simulink model "HEV_Simu_V1_1_RT"  (R2018a)
settings: Solver=ode23s  StartTime=0.0  StopTime=660  FixedStep=0.001  EnableMultiTasking=on
PreLoadFcn:
  | HevSimuVccWs_V1_PreLoad
StartFcn:
  | tic
StopFcn:
  | toc
  | disp(['実時間の' num2str(max(tout)/toc) '倍速'])
model workspace (MAT data in the model file):
  Var = 0
undefined symbols (not defined in the file or in its folder): canChannel
libraries: canmsglib x55, canlib x35, simulink x2, sldrtlib x1
(part 3 of 4)

== system HEV_Simu_V1_1_RT/Controller/CtrlStrct_VNT_Level_2/VNT_Level_2_CAN/Motor_Ctrl/MotorCtrl_PwtrCAN Tx ==
  note: Function of CAN transmit
      | ・conversion fromCAN application signal to signal of CAN message
  note: Motor Control
  note: CAN transmit
  IMotorCtrl_PwtrCAN_Tx_Apli : Inport
  Bus Creator1 : BusCreator  Inputs=1
  Bus Selector1 : BusSelector  OutputSignals=MtrCtrl_Motor_regen_torque_available,MtrCtrl_Motor_torque_actual,MtrCtrl_Motor_torque_available
  MotorCtrl_PwtrCAN Pack : canmsglib/CAN Pack  CANdbFile=HEV_CANDB.dbc  MsgList=MotorCtrl_PwtrCAN_Tx  MsgName=MotorCtrl_PwtrCAN_Tx  MsgIDType=Extended (29-bit identifier)  MsgIdentifier=218058883  MsgLength=8  SignalInfo=MtrCtrl_Motor_regen_torque_avail$32$16$1$1$1$0$1.000000e-02$0$-300$300$#MtrCtrl_Motor_torque_actual$0$16$1$1$1$0$1.000000e-02$0$-300$300$#MtrCtrl_Motor_torque_available$16$16$1$1$1$0$1.000000e-02$0$-300$300$#  NSignals=3  StartBits=str2num('[int32(32);int32(0);int32(16)]')  SignalSizes=str2num('[int32(16);int32(16);int32(16)]')  ByteOrders=str2num('[int32(1);int32(1);int32(1)]')  DataTypes=str2num('[int32(1);int32(1);int32(1)]')  MultiplexTypes=str2num('[int32(1);int32(1);int32(1)]')  MultiplexValues=str2num('[double(0);double(0);double(0)]')  Factors=str2num('[double(1.000000e-02);double(1.000000e-02);double(1.000000e-02)]')  Offsets=str2num('[double(0);double(0);double(0)]')  Minimums=str2num('[double(-300);double(-300);double(-300)]')  Maximums=str2num('[double(300);double(300);double(300)]')  Remote=off  ApplyMinMax=off  BusOutput=off
      settings: AttributesFormatString=<CANdbFile = %<CANdbFile>>  SourceProductName=Simulink Real-Time  SourceProductBaseCode=XP  DataFormat=CANdb specified signals
  MotorCtrl_PwtrCAN Transmit : canlib/CAN Transmit  BlockHandle=19377.0016  DeviceMenu=Vector CANcaseXL 1 (Channel 1)  Device=Vector CANcaseXL 1 (Channel 1)  ObjConstructor=canChannel('Vector','CANcaseXL 1',1)  EnablePeriodicTransmit=on  MessagePeriod=0.01
      settings: AttributesFormatString=<MessagePeriod = %<MessagePeriod>>  SourceProductName=Vehicle Network Toolbox  SourceProductBaseCode=VN
  MotorCtrl_PwtrCAN_Tx_0CFF5083 : Outport
  wires:
  Bus Selector1/2 -> MotorCtrl_PwtrCAN Pack/2  "<MtrCtrl_Motor_torque_actual>"
  Bus Creator1/1 -> MotorCtrl_PwtrCAN Transmit/1, MotorCtrl_PwtrCAN_Tx_0CFF5083/1  "MotorCtrl_PwtrCAN_Tx"
  Bus Selector1/3 -> MotorCtrl_PwtrCAN Pack/3  "<MtrCtrl_Motor_torque_available>"
  MotorCtrl_PwtrCAN Pack/1 -> Bus Creator1/1  "MotorCtrl_PwtrCAN_Tx_0CFF5083"
  IMotorCtrl_PwtrCAN_Tx_Apli/1 -> Bus Selector1/1
  Bus Selector1/1 -> MotorCtrl_PwtrCAN Pack/1  "<MtrCtrl_Motor_regen_torque_available>"

== system HEV_Simu_V1_1_RT/Controller/CtrlStrct_VNT_Level_2/VNT_Level_2_CAN/Motor_Ctrl/MotorCtrl_PwtrCAN_Rx ==
  note: Function of CAN receive
      | ・CAN message selection
      | ・conversion from CAN signal to CAN application signal with bus object
  note: Motor Control
  note: CAN receive
  PwtrCAN : Inport
  Bus Creator7 : BusCreator  Inputs=3
  Bus Selector3 : BusSelector  OutputSignals=HEV_Ctrl_PwtrCAN_Tx_0CFF2082
  Bus Selector4 : BusSelector  OutputSignals=EngineCtrl_PwtrCAN_Tx_0CFF3000
  Bus Selector5 : BusSelector  OutputSignals=TransmCtrl_PwtrCAN_Tx_0CFF4003
  MotorCtrl_PwtrCAN Receive : canlib/CAN Receive  BlockHandle=19439.0016  DeviceMenu=Vector CANcaseXL 1 (Channel 2)  Device=Vector CANcaseXL 1 (Channel 2)  ObjConstructor=canChannel('Vector','CANcaseXL 1',2)  EnableStandardIDsFilter=off  StandardIDs=0  EnableExtendedIDsFilter=off  ExtendedIDs=0  SampleTime=0.01  MsgsPerTimestep=all  StdIDsCombo=Allow all  ExtIDsCombo=Allow all  InternalFilterUpdateStatus=on  BusOutput=off
      settings: AttributesFormatString=<SampleTime = %<SampleTime>>  SourceProductName=Vehicle Network Toolbox  SourceProductBaseCode=VN
  MotorCtrl_PwtrCAN_Receive_10ms : Subsystem
  Rate Transition1 : RateTransition  Deterministic=off
      settings: AttributesFormatString=<Deterministic=%<Deterministic>>
  Terminator : Terminator
  Terminator1 : Terminator
  Terminator2 : Terminator
  MotorCtrl_PwtrCAN_Rx : Outport
  wires:
  PwtrCAN/1 -> Bus Selector4/1, Bus Selector3/1, Bus Selector5/1
  Bus Creator7/1 -> Rate Transition1/1
  Rate Transition1/1 -> MotorCtrl_PwtrCAN_Rx/1  "MotorCtrl_PwtrCAN_Rx"
  Bus Selector5/1 -> Terminator/1  "<TransmCtrl_PwtrCAN_Tx_0CFF4003>"
  Bus Selector3/1 -> Terminator1/1  "<HEV_Ctrl_PwtrCAN_Tx_0CFF2082>"
  Bus Selector4/1 -> Terminator2/1  "<EngineCtrl_PwtrCAN_Tx_0CFF3000>"
  MotorCtrl_PwtrCAN_Receive_10ms/1(TmCtrl_Clutch_position) -> Bus Creator7/1
  MotorCtrl_PwtrCAN_Receive_10ms/2(HEVCtrl_Motor_torque_request) -> Bus Creator7/2
  MotorCtrl_PwtrCAN_Receive_10ms/3(EngCtrl_Engine_speed) -> Bus Creator7/3
  MotorCtrl_PwtrCAN Receive/2 -> MotorCtrl_PwtrCAN_Receive_10ms/1(PwtrCAN_Msg)
  MotorCtrl_PwtrCAN Receive/1 -> MotorCtrl_PwtrCAN_Receive_10ms/Trigger

== system HEV_Simu_V1_1_RT/Controller/CtrlStrct_VNT_Level_2/VNT_Level_2_CAN/NAVI/NAVI_CAN_Rx ==
  note: CAN receive
  note: Navigation
  InfoCAN : Inport
  Bus Creator : BusCreator  Inputs=1  OutDataTypeStr=Bus: NAVI_InfoCAN_Rx_Bus
      settings: AttributesFormatString=<%<OutDataTypeStr>>
  Bus Selector1 : BusSelector  OutputSignals=Gateway_InfoCAN_Tx_0CFFC485
  NAVI_InfoCAN Receive : canlib/CAN Receive  BlockHandle=19512.0016  DeviceMenu=Vector CANcaseXL 1 (Channel 2)  Device=Vector CANcaseXL 1 (Channel 2)  ObjConstructor=canChannel('Vector','CANcaseXL 1',2)  EnableStandardIDsFilter=off  StandardIDs=0  EnableExtendedIDsFilter=off  ExtendedIDs=0  SampleTime=0.1  MsgsPerTimestep=all  StdIDsCombo=Allow all  ExtIDsCombo=Allow all  InternalFilterUpdateStatus=on  BusOutput=off
      settings: AttributesFormatString=<SampleTime = %<SampleTime>>  SourceProductName=Vehicle Network Toolbox  SourceProductBaseCode=VN
  NAVI_InfoCAN_Receive_100ms : Subsystem
  Rate Transition1 : RateTransition  Deterministic=off
      settings: AttributesFormatString=<Deterministic=%<Deterministic>>
  Terminator : Terminator
  NAVI_InfoCAN_Rx : Outport
  wires:
  Rate Transition1/1 -> NAVI_InfoCAN_Rx/1  "NAVI_InfoCAN_Rx"
  InfoCAN/1 -> Bus Selector1/1
  Bus Selector1/1 -> Terminator/1  "<Gateway_InfoCAN_Tx_0CFFC485>"
  NAVI_InfoCAN Receive/2 -> NAVI_InfoCAN_Receive_100ms/1(InfoCAN_Msg)
  NAVI_InfoCAN Receive/1 -> NAVI_InfoCAN_Receive_100ms/Trigger
  Bus Creator/1 -> Rate Transition1/1
  NAVI_InfoCAN_Receive_100ms/1(BrkCtrl_Vehicle_speed) -> Bus Creator/1

== system HEV_Simu_V1_1_RT/Controller/CtrlStrct_VNT_Level_2/VNT_Level_2_CAN/NAVI/NAVI_CAN_Tx ==
  note: CAN transmit
  note: Navigation
  NAVI_InfoCAN_Tx_Apli : Inport
  Bus Creator1 : BusCreator  Inputs=1
  Bus Selector3 : BusSelector  OutputSignals=NAVI_Home_around_status,NAVI_Road_information
  NAVI_InfoCAN Pack : canmsglib/CAN Pack  CANdbFile=HEV_CANDB.dbc  MsgList=NAVI_InfoCAN_Tx  MsgName=NAVI_InfoCAN_Tx  MsgIDType=Extended (29-bit identifier)  MsgIdentifier=218083356  MsgLength=8  SignalInfo=NAVI_Home_around_status$16$16$1$2$1$0$1$0$0$65535$#NAVI_Road_information$0$16$1$2$1$0$1$0$0$65535$#  NSignals=2  StartBits=str2num('[int32(16);int32(0)]')  SignalSizes=str2num('[int32(16);int32(16)]')  ByteOrders=str2num('[int32(1);int32(1)]')  DataTypes=str2num('[int32(2);int32(2)]')  MultiplexTypes=str2num('[int32(1);int32(1)]')  MultiplexValues=str2num('[double(0);double(0)]')  Factors=str2num('[double(1);double(1)]')  Offsets=str2num('[double(0);double(0)]')  Minimums=str2num('[double(0);double(0)]')  Maximums=str2num('[double(65535);double(65535)]')  Remote=off  ApplyMinMax=off  BusOutput=off
      settings: AttributesFormatString=<CANdbFile = %<CANdbFile>>  SourceProductName=Simulink Real-Time  SourceProductBaseCode=XP  DataFormat=CANdb specified signals
  NAVI_InfoCAN Transmit : canlib/CAN Transmit  BlockHandle=20931.0017  DeviceMenu=Vector CANcaseXL 1 (Channel 1)  Device=Vector CANcaseXL 1 (Channel 1)  ObjConstructor=canChannel('Vector','CANcaseXL 1',1)  EnablePeriodicTransmit=on  MessagePeriod=0.1
      settings: AttributesFormatString=<MessagePeriod = %<MessagePeriod>>  SourceProductName=Vehicle Network Toolbox  SourceProductBaseCode=VN
  NAVI_InfoCAN_Tx : Outport
  wires:
  Bus Creator1/1 -> NAVI_InfoCAN_Tx/1  "NAVI_InfoCAN_Tx"
  Bus Selector3/1 -> NAVI_InfoCAN Pack/1  "<NAVI_Home_around_status>"
  NAVI_InfoCAN Pack/1 -> NAVI_InfoCAN Transmit/1, Bus Creator1/1  "NAVI_InfoCAN_Tx_0CFFB01C"
  Bus Selector3/2 -> NAVI_InfoCAN Pack/2  "<NAVI_Road_information>"
  NAVI_InfoCAN_Tx_Apli/1 -> Bus Selector3/1

== system HEV_Simu_V1_1_RT/Controller/CtrlStrct_VNT_Level_2/VNT_Level_2_CAN/Radar/Radar_CAN_Rx ==
  note: Function of CAN receive
      | ・CAN message selection
      | ・conversion from CAN signal to CAN application signal with bus object
  note: Radar Detection
  note: CAN receive
  InfoCAN : Inport
  Bus Creator : BusCreator  Inputs=1
  Bus Selector1 : BusSelector  OutputSignals=Gateway_InfoCAN_Tx_0CFFC485
  Radar_InfoCAN Receive : canlib/CAN Receive  BlockHandle=20997.0016  DeviceMenu=Vector CANcaseXL 1 (Channel 2)  Device=Vector CANcaseXL 1 (Channel 2)  ObjConstructor=canChannel('Vector','CANcaseXL 1',2)  EnableStandardIDsFilter=off  StandardIDs=0  EnableExtendedIDsFilter=off  ExtendedIDs=0  SampleTime=0.1  MsgsPerTimestep=all  StdIDsCombo=Allow all  ExtIDsCombo=Allow all  InternalFilterUpdateStatus=on  BusOutput=off
      settings: AttributesFormatString=<SampleTime = %<SampleTime>>  SourceProductName=Vehicle Network Toolbox  SourceProductBaseCode=VN
  Radar_InfoCAN_Receive_100ms : Subsystem
  Rate Transition1 : RateTransition  Deterministic=off
      settings: AttributesFormatString=<Deterministic=%<Deterministic>>
  Terminator : Terminator
  Radar_InfoCAN_Rx : Outport
  wires:
  Rate Transition1/1 -> Radar_InfoCAN_Rx/1  "Radar_InfoCAN_Rx"
  Bus Creator/1 -> Rate Transition1/1
  InfoCAN/1 -> Bus Selector1/1
  Bus Selector1/1 -> Terminator/1  "<Gateway_InfoCAN_Tx_0CFFC485>"
  Radar_InfoCAN_Receive_100ms/1(BrkCtrl_Vehicle_speed) -> Bus Creator/1
  Radar_InfoCAN Receive/2 -> Radar_InfoCAN_Receive_100ms/1(InfoCAN_Msg)
  Radar_InfoCAN Receive/1 -> Radar_InfoCAN_Receive_100ms/Trigger

== system HEV_Simu_V1_1_RT/Controller/CtrlStrct_VNT_Level_2/VNT_Level_2_CAN/Radar/Radar_CAN_Tx ==
  note: Radar Detection
  note: CAN transmit
  note: Function of CAN transmit
      | ・conversion fromCAN application signal to signal of CAN message
  Radar_InfoCAN_Tx_Apli : Inport
  Bus Creator1 : BusCreator  Inputs=1
  Bus Selector3 : BusSelector  OutputSignals=Radar_Relative_distance,Radar_Relative_velocity
  Radar_InfoCAN Pack : canmsglib/CAN Pack  CANdbFile=HEV_CANDB.dbc  MsgList=Radar_InfoCAN_Tx  MsgName=Radar_InfoCAN_Tx  MsgIDType=Extended (29-bit identifier)  MsgIdentifier=218038400  MsgLength=8  SignalInfo=Radar_Relative_distance$0$16$1$2$1$0$1.000000e-02$0$0$500$#Radar_Relative_velocity$16$16$1$1$1$0$1.000000e-02$0$-50$50$#  NSignals=2  StartBits=str2num('[int32(0);int32(16)]')  SignalSizes=str2num('[int32(16);int32(16)]')  ByteOrders=str2num('[int32(1);int32(1)]')  DataTypes=str2num('[int32(2);int32(1)]')  MultiplexTypes=str2num('[int32(1);int32(1)]')  MultiplexValues=str2num('[double(0);double(0)]')  Factors=str2num('[double(1.000000e-02);double(1.000000e-02)]')  Offsets=str2num('[double(0);double(0)]')  Minimums=str2num('[double(0);double(-50)]')  Maximums=str2num('[double(500);double(50)]')  Remote=off  ApplyMinMax=off  BusOutput=off
      settings: AttributesFormatString=<CANdbFile = %<CANdbFile>>  SourceProductName=Simulink Real-Time  SourceProductBaseCode=XP  DataFormat=CANdb specified signals
  Radar_InfoCAN Transmit : canlib/CAN Transmit  BlockHandle=21025.0016  DeviceMenu=Vector CANcaseXL 1 (Channel 1)  Device=Vector CANcaseXL 1 (Channel 1)  ObjConstructor=canChannel('Vector','CANcaseXL 1',1)  EnablePeriodicTransmit=on  MessagePeriod=0.1
      settings: AttributesFormatString=<MessagePeriod = %<MessagePeriod>>  SourceProductName=Vehicle Network Toolbox  SourceProductBaseCode=VN
  Radar_InfoCAN_Tx : Outport
  wires:
  Bus Creator1/1 -> Radar_InfoCAN_Tx/1  "Radar_InfoCAN_Tx"
  Radar_InfoCAN_Tx_Apli/1 -> Bus Selector3/1
  Radar_InfoCAN Pack/1 -> Bus Creator1/1, Radar_InfoCAN Transmit/1  "Radar_InfoCAN_Tx_0CFF0080"
  Bus Selector3/2 -> Radar_InfoCAN Pack/2  "<Radar_Relative_velocity>"
  Bus Selector3/1 -> Radar_InfoCAN Pack/1  "<Radar_Relative_distance>"

== system HEV_Simu_V1_1_RT/Controller/CtrlStrct_VNT_Level_2/VNT_Level_2_CAN/Steer_Ctrl/SteerCtrl_VehCAN Tx ==
  note: Steering Control
  note: Function of CAN transmit
      | ・conversion fromCAN application signal to signal of CAN message
  note: CAN transmit
  SteerCtrl_VehCAN_Tx_Apli : Inport
  Bus Creator1 : BusCreator  Inputs=1
  Bus Selector1 : BusSelector  OutputSignals=StrgCtrl_Steer_angle
  SteerCtrl_VehCAN Pack : canmsglib/CAN Pack  CANdbFile=HEV_CANDB.dbc  MsgList=SteerCtrl_VehCAN_Tx  MsgName=SteerCtrl_VehCAN_Tx  MsgIDType=Extended (29-bit identifier)  MsgIdentifier=218066963  MsgLength=8  SignalInfo=StrgCtrl_Steer_angle$0$16$1$1$1$0$3.125000e-02$0$-720$720$#  NSignals=1  StartBits=str2num('[int32(0)]')  SignalSizes=str2num('[int32(16)]')  ByteOrders=str2num('[int32(1)]')  DataTypes=str2num('[int32(1)]')  MultiplexTypes=str2num('[int32(1)]')  MultiplexValues=str2num('[double(0)]')  Factors=str2num('[double(3.125000e-02)]')  Offsets=str2num('[double(0)]')  Minimums=str2num('[double(-720)]')  Maximums=str2num('[double(720)]')  Remote=off  ApplyMinMax=off  BusOutput=off
      settings: AttributesFormatString=<CANdbFile = %<CANdbFile>>  SourceProductName=Simulink Real-Time  SourceProductBaseCode=XP  DataFormat=CANdb specified signals
  SteerCtrl_VehCAN Transmit : canlib/CAN Transmit  BlockHandle=21054.0016  DeviceMenu=Vector CANcaseXL 1 (Channel 1)  Device=Vector CANcaseXL 1 (Channel 1)  ObjConstructor=canChannel('Vector','CANcaseXL 1',1)  EnablePeriodicTransmit=on  MessagePeriod=0.05
      settings: AttributesFormatString=<MessagePeriod = %<MessagePeriod>>  SourceProductName=Vehicle Network Toolbox  SourceProductBaseCode=VN
  SteerCtrl_VehCAN_Tx : Outport
  wires:
  SteerCtrl_VehCAN Pack/1 -> SteerCtrl_VehCAN Transmit/1, Bus Creator1/1  "SteerCtrl_VehCAN_Tx_0CFF7013"
  Bus Selector1/1 -> SteerCtrl_VehCAN Pack/1  "<StrgCtrl_Steer_angle>"
  SteerCtrl_VehCAN_Tx_Apli/1 -> Bus Selector1/1
  Bus Creator1/1 -> SteerCtrl_VehCAN_Tx/1  "SteerCtrl_VehCAN_Tx"

== system HEV_Simu_V1_1_RT/Controller/CtrlStrct_VNT_Level_2/VNT_Level_2_CAN/Steer_Ctrl/SteerCtrl_VehCAN_Rx ==
  note: Steering Control
  note: Function of CAN receive
      | ・CAN message selection
      | ・conversion from CAN signal to CAN application signal with bus object
  note: CAN receive
  In1 : Inport
  Bus Creator : BusCreator  Inputs=1
  Bus Selector7 : BusSelector  OutputSignals=BrakeCtrl_VehCAN_Tx_0CFF600B
  Rate Transition1 : RateTransition  Deterministic=off
      settings: AttributesFormatString=<Deterministic=%<Deterministic>>
  SteerCtrl_VehCAN Receive : canlib/CAN Receive  BlockHandle=21070.0016  DeviceMenu=Vector CANcaseXL 1 (Channel 2)  Device=Vector CANcaseXL 1 (Channel 2)  ObjConstructor=canChannel('Vector','CANcaseXL 1',2)  EnableStandardIDsFilter=off  StandardIDs=0  EnableExtendedIDsFilter=off  ExtendedIDs=0  SampleTime=0.05  MsgsPerTimestep=all  StdIDsCombo=Allow all  ExtIDsCombo=Allow all  InternalFilterUpdateStatus=on  BusOutput=off
      settings: AttributesFormatString=<SampleTime = %<SampleTime>>  SourceProductName=Vehicle Network Toolbox  SourceProductBaseCode=VN
  SteerCtrl_VehCAN_Receive50ms : Subsystem
  Terminator : Terminator
  SteerCtrl_VehCAN_Rx : Outport
  wires:
  In1/1 -> Bus Selector7/1
  Bus Creator/1 -> Rate Transition1/1
  Rate Transition1/1 -> SteerCtrl_VehCAN_Rx/1  "SteerCtrl_VehCAN_Rx"
  Bus Selector7/1 -> Terminator/1  "<BrakeCtrl_VehCAN_Tx_0CFF600B>"
  SteerCtrl_VehCAN_Receive50ms/1(BrkCtrl_Vehicle_speed) -> Bus Creator/1
  SteerCtrl_VehCAN Receive/1 -> SteerCtrl_VehCAN_Receive50ms/Trigger
  SteerCtrl_VehCAN Receive/2 -> SteerCtrl_VehCAN_Receive50ms/1(VehCAN_Msg)

== system HEV_Simu_V1_1_RT/Controller/CtrlStrct_VNT_Level_2/VNT_Level_2_CAN/Transms_Ctrl/TransmCtrl_PwtrCAN Tx ==
  note: Function of CAN transmit
      | ・conversion fromCAN application signal to signal of CAN message
  note: Transmission Control
  note: CAN transmit
  TransmCtrl_PwtrCAN_Tx_Apli : Inport
  Bus Creator1 : BusCreator  Inputs=1
  Bus Selector2 : BusSelector  OutputSignals=TmCtrl_Clutch_position,TmCtrl_Gear_position
  TransmCtrl_PwtrCAN Pack : canmsglib/CAN Pack  CANdbFile=HEV_CANDB.dbc  MsgList=TransmCtrl_PwtrCAN_Tx  MsgName=TransmCtrl_PwtrCAN_Tx  MsgIDType=Extended (29-bit identifier)  MsgIdentifier=218054659  MsgLength=8  SignalInfo=TmCtrl_Clutch_position$0$8$1$2$1$0$1.000000e-02$0$0$1$#TmCtrl_Gear_position$8$8$1$2$1$0$1$0$0$5$#  NSignals=2  StartBits=str2num('[int32(0);int32(8)]')  SignalSizes=str2num('[int32(8);int32(8)]')  ByteOrders=str2num('[int32(1);int32(1)]')  DataTypes=str2num('[int32(2);int32(2)]')  MultiplexTypes=str2num('[int32(1);int32(1)]')  MultiplexValues=str2num('[double(0);double(0)]')  Factors=str2num('[double(1.000000e-02);double(1)]')  Offsets=str2num('[double(0);double(0)]')  Minimums=str2num('[double(0);double(0)]')  Maximums=str2num('[double(1);double(5)]')  Remote=off  ApplyMinMax=off  BusOutput=off
      settings: AttributesFormatString=<CANdbFile = %<CANdbFile>>  SourceProductName=Simulink Real-Time  SourceProductBaseCode=XP  DataFormat=CANdb specified signals
  TransmCtrl_PwtrCAN Transmit : canlib/CAN Transmit  BlockHandle=21269.0016  DeviceMenu=Vector CANcaseXL 1 (Channel 1)  Device=Vector CANcaseXL 1 (Channel 1)  ObjConstructor=canChannel('Vector','CANcaseXL 1',1)  EnablePeriodicTransmit=on  MessagePeriod=0.01
      settings: AttributesFormatString=<MessagePeriod = %<MessagePeriod>>  SourceProductName=Vehicle Network Toolbox  SourceProductBaseCode=VN
  TransmCtrl_PwtrCAN_Tx : Outport
  wires:
  TransmCtrl_PwtrCAN_Tx_Apli/1 -> Bus Selector2/1
  TransmCtrl_PwtrCAN Pack/1 -> Bus Creator1/1  "TransmCtrl_PwtrCAN_Tx_0CFF4003"
  Bus Creator1/1 -> TransmCtrl_PwtrCAN Transmit/1, TransmCtrl_PwtrCAN_Tx/1  "TransmCtrl_PwtrCAN_Tx"
  Bus Selector2/2 -> TransmCtrl_PwtrCAN Pack/2  "<TmCtrl_Gear_position>"
  Bus Selector2/1 -> TransmCtrl_PwtrCAN Pack/1  "<TmCtrl_Clutch_position>"

== system HEV_Simu_V1_1_RT/Controller/CtrlStrct_VNT_Level_2/VNT_Level_2_CAN/Transms_Ctrl/TransmCtrl_PwtrCAN_Rx ==
  note: Transmission Control
  note: Function of CAN receive
      | ・CAN message selection
      | ・conversion from CAN signal to CAN application signal with bus object
  note: CAN receive
  PwtrCAN : Inport
  Bus Creator6 : BusCreator  Inputs=2
  Bus Selector3 : BusSelector  OutputSignals=EngineCtrl_PwtrCAN_Tx_0CFF3000
  Bus Selector7 : BusSelector  OutputSignals=Gateway_PwtrCAN_Tx_0CFFC385
  Rate Transition1 : RateTransition  Deterministic=off
      settings: AttributesFormatString=<Deterministic=%<Deterministic>>
  Terminator : Terminator
  Terminator1 : Terminator
  TransmCtrl_PwtrCAN Receive : canlib/CAN Receive  BlockHandle=23424.0016  DeviceMenu=Vector CANcaseXL 1 (Channel 2)  Device=Vector CANcaseXL 1 (Channel 2)  ObjConstructor=canChannel('Vector','CANcaseXL 1',2)  EnableStandardIDsFilter=off  StandardIDs=0  EnableExtendedIDsFilter=off  ExtendedIDs=0  SampleTime=0.01  MsgsPerTimestep=all  StdIDsCombo=Allow all  ExtIDsCombo=Allow all  InternalFilterUpdateStatus=on  BusOutput=off
      settings: AttributesFormatString=<SampleTime = %<SampleTime>>  SourceProductName=Vehicle Network Toolbox  SourceProductBaseCode=VN
  TransmCtrl_PwtrCAN_Receive_10ms : Subsystem
  TransmCtrl_PwtrCAN_Rx : Outport
  wires:
  PwtrCAN/1 -> Bus Selector3/1, Bus Selector7/1
  Rate Transition1/1 -> TransmCtrl_PwtrCAN_Rx/1  "TransmCtrl_PwtrCAN_Rx"
  Bus Creator6/1 -> Rate Transition1/1
  Bus Selector7/1 -> Terminator/1  "<Gateway_PwtrCAN_Tx_0CFFC385>"
  Bus Selector3/1 -> Terminator1/1  "<EngineCtrl_PwtrCAN_Tx_0CFF3000>"
  TransmCtrl_PwtrCAN_Receive_10ms/1(BrkCtrl_Vehicle_speed) -> Bus Creator6/1
  TransmCtrl_PwtrCAN_Receive_10ms/2(EngCtrl_Engine_speed) -> Bus Creator6/2
  TransmCtrl_PwtrCAN Receive/1 -> TransmCtrl_PwtrCAN_Receive_10ms/Trigger
  TransmCtrl_PwtrCAN Receive/2 -> TransmCtrl_PwtrCAN_Receive_10ms/1(PwtrCAN_Msg)

== system HEV_Simu_V1_1_RT/Controller/CtrlStrct_VNT_Level_2/VNT_Level_2_CAN/VM_Ctrl/VM_Ctrl_VehCAN Tx ==
  note: Vehicle Motion Control
  note: Function of CAN transmit
      | ・conversion fromCAN application signal to signal of CAN message
  note: CAN transmit
  VM_Ctrl_VehCAN_Tx_Apli : Inport
  Bus Creator1 : BusCreator  Inputs=1
  Bus Selector3 : BusSelector  OutputSignals=VMCtrl_BrakeForceCmnd,VMCtrl_BrakeForceStatus,VMCtrl_PropTorqCmnd,VMCtrl_PropTorqStatus
  VM_Ctrl_VehCAN Pack : canmsglib/CAN Pack  CANdbFile=HEV_CANDB.dbc  MsgList=VM_Ctrl_VehCAN_Tx  MsgName=VM_Ctrl_VehCAN_Tx  MsgIDType=Extended (29-bit identifier)  MsgIdentifier=218091654  MsgLength=8  SignalInfo=VMCtrl_BrakeTorqCmnd$32$16$1$1$1$0$1.000000e-02$0$-300$300$#VMCtrl_BrakeTorqStatus$24$8$1$2$1$0$1$0$0$7$#VMCtrl_PropTorqCmnd$8$16$1$1$1$0$1.000000e-02$0$-300$300$#VMCtrl_PropTorqStatus$0$8$1$2$1$0$1$0$-Inf$Inf$#  NSignals=4  StartBits=str2num('[int32(32);int32(24);int32(8);int32(0)]')  SignalSizes=str2num('[int32(16);int32(8);int32(16);int32(8)]')  ByteOrders=str2num('[int32(1);int32(1);int32(1);int32(1)]')  DataTypes=str2num('[int32(1);int32(2);int32(1);int32(2)]')  MultiplexTypes=str2num('[int32(1);int32(1);int32(1);int32(1)]')  MultiplexValues=str2num('[double(0);double(0);double(0);double(0)]')  Factors=str2num('[double(1.000000e-02);double(1);double(1.000000e-02);double(1)]')  Offsets=str2num('[double(0);double(0);double(0);double(0)]')  Minimums=str2num('[double(-300);double(0);double(-300);double(-Inf)]')  Maximums=str2num('[double(300);double(7);double(300);double(Inf)]')  Remote=off  ApplyMinMax=off  BusOutput=off
      settings: AttributesFormatString=<CANdbFile = %<CANdbFile>>  SourceProductName=Simulink Real-Time  SourceProductBaseCode=XP  DataFormat=CANdb specified signals
  VM_Ctrl_VehCAN Transmit : canlib/CAN Transmit  BlockHandle=26337.0018  DeviceMenu=Vector CANcaseXL 1 (Channel 1)  Device=Vector CANcaseXL 1 (Channel 1)  ObjConstructor=canChannel('Vector','CANcaseXL 1',1)  EnablePeriodicTransmit=on  MessagePeriod=0.05
      settings: AttributesFormatString=<MessagePeriod = %<MessagePeriod>>  SourceProductName=Vehicle Network Toolbox  SourceProductBaseCode=VN
  VM_Ctrl_VehCAN_Tx : Outport
  wires:
  Bus Selector3/1 -> VM_Ctrl_VehCAN Pack/1  "<VMCtrl_BrakeForceCmnd>"
  Bus Selector3/2 -> VM_Ctrl_VehCAN Pack/2  "<VMCtrl_BrakeForceStatus>"
  Bus Selector3/3 -> VM_Ctrl_VehCAN Pack/3  "<VMCtrl_PropTorqCmnd>"
  VM_Ctrl_VehCAN Pack/1 -> VM_Ctrl_VehCAN Transmit/1, Bus Creator1/1  "VM_Ctrl_VehCAN_Tx_0CFFD086"
  VM_Ctrl_VehCAN_Tx_Apli/1 -> Bus Selector3/1
  Bus Creator1/1 -> VM_Ctrl_VehCAN_Tx/1  "VM_Ctrl_VehCAN_Tx"
  Bus Selector3/4 -> VM_Ctrl_VehCAN Pack/4  "<VMCtrl_PropTorqStatus>"

== system HEV_Simu_V1_1_RT/Controller/CtrlStrct_VNT_Level_2/VNT_Level_2_CAN/VM_Ctrl/VM_Ctrl_VehCAN_Rx ==
  note: Vehicle Motion Control
  note: Function of CAN receive
      | ・CAN message selection
      | ・conversion from CAN signal to CAN application signal with bus object
  note: CAN receive
  In1 : Inport
  Bus Creator : BusCreator  Inputs=1
  Bus Selector7 : BusSelector  OutputSignals=BrakeCtrl_VehCAN_Tx_0CFF600B
  Rate Transition1 : RateTransition  Deterministic=off
      settings: AttributesFormatString=<Deterministic=%<Deterministic>>
  Terminator : Terminator
  VM_Ctrl_VehCAN Receive : canlib/CAN Receive  BlockHandle=26357.0018  DeviceMenu=Vector CANcaseXL 1 (Channel 2)  Device=Vector CANcaseXL 1 (Channel 2)  ObjConstructor=canChannel('Vector','CANcaseXL 1',2)  EnableStandardIDsFilter=off  StandardIDs=0  EnableExtendedIDsFilter=off  ExtendedIDs=0  SampleTime=0.05  MsgsPerTimestep=all  StdIDsCombo=Allow all  ExtIDsCombo=Allow all  InternalFilterUpdateStatus=on  BusOutput=off
      settings: AttributesFormatString=<SampleTime = %<SampleTime>>  SourceProductName=Vehicle Network Toolbox  SourceProductBaseCode=VN
  VM_Ctrl_VehCAN_Receive_50ms : Subsystem
  VM_Ctrl_VehCAN_Rx : Outport
  wires:
  Bus Creator/1 -> Rate Transition1/1
  Rate Transition1/1 -> VM_Ctrl_VehCAN_Rx/1  "VM_Ctrl_VehCAN_Rx"
  In1/1 -> Bus Selector7/1
  Bus Selector7/1 -> Terminator/1  "<BrakeCtrl_VehCAN_Tx_0CFF600B>"
  VM_Ctrl_VehCAN_Receive_50ms/1(BrkCtrl_Vehicle_speed) -> Bus Creator/1
  VM_Ctrl_VehCAN Receive/1 -> VM_Ctrl_VehCAN_Receive_50ms/Trigger
  VM_Ctrl_VehCAN Receive/2 -> VM_Ctrl_VehCAN_Receive_50ms/1(VehCAN_Msg)

== system HEV_Simu_V1_1_RT/Controller/CtrlStrct_VNT_Level_2/VNT_Level_2_CAN/Battery_Ctrl/BatteryCtrl_PwtrCAN_Rx/BatteryCtrl_PwtrCAN_Receive_50ms ==
  PwtrCAN_Msg : Inport
  function : TriggerPort  TriggerType=function-call  VariantControl=Variant
  BatteryCtrl_PwtrCAN Unpack : canmsglib/CAN Unpack  CANdbFile=HEV_CANDB.dbc  MsgList=HEV_Ctrl_PwtrCAN_Tx_1  MsgName=HEV_Ctrl_PwtrCAN_Tx_1  MsgIDType=Extended (29-bit identifier)  MsgIdentifier=218046594  MsgLength=8  SignalInfo=HEVCtrl_Engine_torque_request$0$16$1$1$1$0$1.562500e-02$0$-300$300$#HEVCtrl_Motor_torque_request$16$16$1$1$1$0$1.562500e-02$0$-300$300$#HEVCtrl_Regen_brake_torque_actua$48$16$1$1$1$0$6.250000e-02$0$-300$3000$#HEVCtrl_Regen_brake_torque_avail$32$16$1$1$1$0$6.250000e-02$0$-300$3000$#  NSignals=4  IDPort=off  TimestampPort=off  ErrorPort=off  RemotePort=off  LengthPort=off  StatusPort=off  StartBits=str2num('[int32(0);int32(16);int32(48);int32(32)]')  SignalSizes=str2num('[int32(16);int32(16);int32(16);int32(16)]')  ByteOrders=str2num('[int32(1);int32(1);int32(1);int32(1)]')  DataTypes=str2num('[int32(1);int32(1);int32(1);int32(1)]')  MultiplexTypes=str2num('[int32(1);int32(1);int32(1);int32(1)]')  MultiplexValues=str2num('[double(0);double(0);double(0);double(0)]')  Factors=str2num('[double(1.562500e-02);double(1.562500e-02);double(6.250000e-02);double(6.250000e-02)]')  Offsets=str2num('[double(0);double(0);double(0);double(0)]')  Minimums=str2num('[double(-300);double(-300);double(-300);double(-300)]')  Maximums=str2num('[double(300);double(300);double(3000);double(3000)]')  ApplyMinMax=off
      settings: AttributesFormatString=<CANdbFile = %<CANdbFile>>  SourceProductName=Simulink Real-Time  SourceProductBaseCode=XP  DataFormat=CANdb specified signals
  Signal Specification : SignalSpecification
  Terminator1 : Terminator
  Terminator2 : Terminator
  Terminator3 : Terminator
  HEVCtrl_Motor_torque_request : Outport
  wires:
  BatteryCtrl_PwtrCAN Unpack/3 -> Terminator2/1
  BatteryCtrl_PwtrCAN Unpack/4 -> Terminator3/1
  BatteryCtrl_PwtrCAN Unpack/2 -> Signal Specification/1  "PwtrCAN_HEVCtrl_Motor_torque_request"
  BatteryCtrl_PwtrCAN Unpack/1 -> Terminator1/1
  PwtrCAN_Msg/1 -> BatteryCtrl_PwtrCAN Unpack/1
  Signal Specification/1 -> HEVCtrl_Motor_torque_request/1  "HEVCtrl_Motor_torque_request"

== system HEV_Simu_V1_1_RT/Controller/CtrlStrct_VNT_Level_2/VNT_Level_2_CAN/Body_Ctrl/BodyCtrl_VehCAN_Rx/BodyCtrl_VehCAN_Receive_50ms ==
  VehCAN_Msg : Inport
  function : TriggerPort  TriggerType=function-call  VariantControl=Variant
  BodyCtrl_VehCAN Unpack : canmsglib/CAN Unpack  CANdbFile=HEV_CANDB.dbc  MsgList=BrakeCtrl_VehCAN_Tx  MsgName=BrakeCtrl_VehCAN_Tx  MsgIDType=Extended (29-bit identifier)  MsgIdentifier=218062859  MsgLength=8  SignalInfo=BrkCtrl_Regen_brake_torque_reque$16$16$1$1$1$0$1.000000e-02$0$-300$300$#BrkCtrl_Vehicle_speed$0$16$1$2$1$0$1.000000e-01$0$0$180$#  NSignals=2  IDPort=off  TimestampPort=off  ErrorPort=off  RemotePort=off  LengthPort=off  StatusPort=off  StartBits=str2num('[int32(16);int32(0)]')  SignalSizes=str2num('[int32(16);int32(16)]')  ByteOrders=str2num('[int32(1);int32(1)]')  DataTypes=str2num('[int32(1);int32(2)]')  MultiplexTypes=str2num('[int32(1);int32(1)]')  MultiplexValues=str2num('[double(0);double(0)]')  Factors=str2num('[double(1.000000e-02);double(1.000000e-01)]')  Offsets=str2num('[double(0);double(0)]')  Minimums=str2num('[double(-300);double(0)]')  Maximums=str2num('[double(300);double(180)]')  ApplyMinMax=off
      settings: AttributesFormatString=<CANdbFile = %<CANdbFile>>  SourceProductName=Simulink Real-Time  SourceProductBaseCode=XP  DataFormat=CANdb specified signals
  BodyCtrl_VehCAN Unpack2 : canmsglib/CAN Unpack  CANdbFile=HEV_CANDB.dbc  MsgList=Gateway_VehCAN_Tx_2  MsgName=Gateway_VehCAN_Tx_2  MsgIDType=Extended (29-bit identifier)  MsgIdentifier=218087813  MsgLength=8  SignalInfo=EngCtrl_Engine_speed_G$0$16$1$2$1$0$1.250000e-01$0$0$8192$#HEV_IdleStopCtrl_preparation_r_G$24$1$1$2$1$0$1$0$0$1$#HEV_IdleStopCtrl_request_G$25$1$1$2$1$0$1$0$0$1$#HEV_IdleStopCtrl_status_G$26$1$1$2$1$0$1$0$0$1$#TmCtrl_Gear_position_G$16$8$1$2$1$0$1$0$0$5$#  NSignals=5  IDPort=off  TimestampPort=off  ErrorPort=off  RemotePort=off  LengthPort=off  StatusPort=off  StartBits=str2num('[int32(0);int32(24);int32(25);int32(26);int32(16)]')  SignalSizes=str2num('[int32(16);int32(1);int32(1);int32(1);int32(8)]')  ByteOrders=str2num('[int32(1);int32(1);int32(1);int32(1);int32(1)]')  DataTypes=str2num('[int32(2);int32(2);int32(2);int32(2);int32(2)]')  MultiplexTypes=str2num('[int32(1);int32(1);int32(1);int32(1);int32(1)]')  MultiplexValues=str2num('[double(0);double(0);double(0);double(0);double(0)]')  Factors=str2num('[double(1.250000e-01);double(1);double(1);double(1);double(1)]')  Offsets=str2num('[double(0);double(0);double(0);double(0);double(0)]')  Minimums=str2num('[double(0);double(0);double(0);double(0);double(0)]')  Maximums=str2num('[double(8192);double(1);double(1);double(1);double(5)]')  ApplyMinMax=off
      settings: AttributesFormatString=<CANdbFile = %<CANdbFile>>  SourceProductName=Simulink Real-Time  SourceProductBaseCode=XP  DataFormat=CANdb specified signals
  Signal Specification : SignalSpecification
  Signal Specification1 : SignalSpecification
  Signal Specification2 : SignalSpecification
  Terminator{3..6} (4 alike) : Terminator
  BrkCtrl_Vehicle_speed : Outport
  EngCtrl_Engine_speed : Outport  Port=2
  HEVCtrl_IdleStop_status : Outport  Port=3
  wires:
  VehCAN_Msg/1 -> BodyCtrl_VehCAN Unpack2/1, BodyCtrl_VehCAN Unpack/1
  BodyCtrl_VehCAN Unpack2/2 -> Terminator3/1
  BodyCtrl_VehCAN Unpack2/3 -> Terminator5/1
  BodyCtrl_VehCAN Unpack/1 -> Terminator4/1  "VehCAN_BrkCtrl_Regen_brake_torque_request"
  BodyCtrl_VehCAN Unpack2/5 -> Terminator6/1
  BodyCtrl_VehCAN Unpack2/1 -> Signal Specification1/1  "VehCAN_EngCtrl_Engine_speed"
  BodyCtrl_VehCAN Unpack2/4 -> Signal Specification2/1  "VehCAN_HEVCtrl_IdleStop_status"
  BodyCtrl_VehCAN Unpack/2 -> Signal Specification/1  "VehCAN_BrkCtrl_Vehicle_speed"
  Signal Specification/1 -> BrkCtrl_Vehicle_speed/1  "BrkCtrl_Vehicle_speed"
  Signal Specification1/1 -> EngCtrl_Engine_speed/1  "EngCtrl_Engine_speed"
  Signal Specification2/1 -> HEVCtrl_IdleStop_status/1  "HEVCtrl_IdleStop_status"

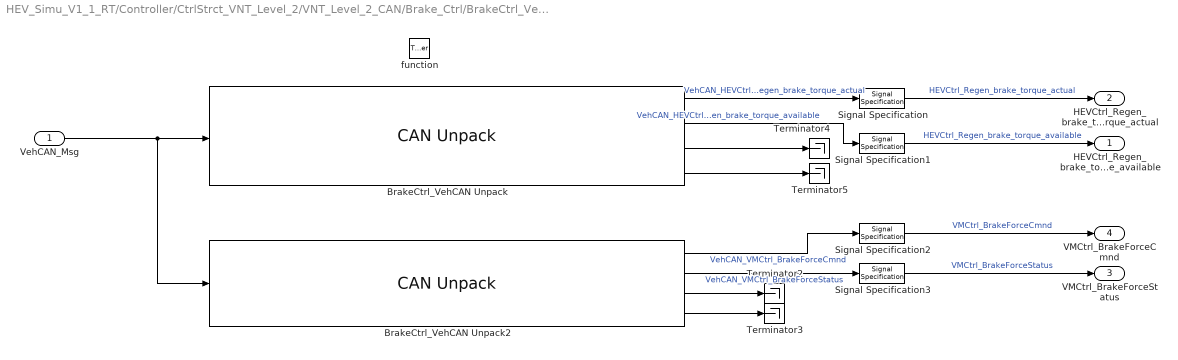
== system HEV_Simu_V1_1_RT/Controller/CtrlStrct_VNT_Level_2/VNT_Level_2_CAN/Brake_Ctrl/BrakeCtrl_VehCAN_Rx/BrakeCtrl_VehCAN_Receive_10ms ==
  VehCAN_Msg : Inport
  function : TriggerPort  TriggerType=function-call  VariantControl=Variant
  BrakeCtrl_VehCAN Unpack : canmsglib/CAN Unpack  CANdbFile=HEV_CANDB.dbc  MsgList=Gateway_VehCAN_Tx_1  MsgName=Gateway_VehCAN_Tx_1  MsgIDType=Extended (29-bit identifier)  MsgIdentifier=218087557  MsgLength=8  SignalInfo=HEVCtrl_Regen_brake_torque_act_G$48$16$1$1$1$0$6.250000e-02$0$-300$3000$#HEVCtrl_Regen_brake_torque_ave_G$32$16$1$1$1$0$6.250000e-02$0$-300$3000$#Radar_Relative_distance_G$0$16$1$2$1$0$1.000000e-02$0$0$500$#Radar_Relative_velocity_G$16$16$1$1$1$0$1.000000e-02$0$-50$50$#  NSignals=4  IDPort=off  TimestampPort=off  ErrorPort=off  RemotePort=off  LengthPort=off  StatusPort=off  StartBits=str2num('[int32(48);int32(32);int32(0);int32(16)]')  SignalSizes=str2num('[int32(16);int32(16);int32(16);int32(16)]')  ByteOrders=str2num('[int32(1);int32(1);int32(1);int32(1)]')  DataTypes=str2num('[int32(1);int32(1);int32(2);int32(1)]')  MultiplexTypes=str2num('[int32(1);int32(1);int32(1);int32(1)]')  MultiplexValues=str2num('[double(0);double(0);double(0);double(0)]')  Factors=str2num('[double(6.250000e-02);double(6.250000e-02);double(1.000000e-02);double(1.000000e-02)]')  Offsets=str2num('[double(0);double(0);double(0);double(0)]')  Minimums=str2num('[double(-300);double(-300);double(0);double(-50)]')  Maximums=str2num('[double(3000);double(3000);double(500);double(50)]')  ApplyMinMax=off
      settings: AttributesFormatString=<CANdbFile = %<CANdbFile>>  SourceProductName=Simulink Real-Time  SourceProductBaseCode=XP  DataFormat=CANdb specified signals
  BrakeCtrl_VehCAN Unpack2 : canmsglib/CAN Unpack  CANdbFile=HEV_CANDB.dbc  MsgList=VM_Ctrl_VehCAN_Tx  MsgName=VM_Ctrl_VehCAN_Tx  MsgIDType=Extended (29-bit identifier)  MsgIdentifier=218091654  MsgLength=8  SignalInfo=VMCtrl_BrakeTorqCmnd$32$16$1$1$1$0$1.000000e-02$0$-300$300$#VMCtrl_BrakeTorqStatus$24$8$1$2$1$0$1$0$0$7$#VMCtrl_PropTorqCmnd$8$16$1$1$1$0$1.000000e-02$0$-300$300$#VMCtrl_PropTorqStatus$0$8$1$2$1$0$1$0$-Inf$Inf$#  NSignals=4  IDPort=off  TimestampPort=off  ErrorPort=off  RemotePort=off  LengthPort=off  StatusPort=off  StartBits=str2num('[int32(32);int32(24);int32(8);int32(0)]')  SignalSizes=str2num('[int32(16);int32(8);int32(16);int32(8)]')  ByteOrders=str2num('[int32(1);int32(1);int32(1);int32(1)]')  DataTypes=str2num('[int32(1);int32(2);int32(1);int32(2)]')  MultiplexTypes=str2num('[int32(1);int32(1);int32(1);int32(1)]')  MultiplexValues=str2num('[double(0);double(0);double(0);double(0)]')  Factors=str2num('[double(1.000000e-02);double(1);double(1.000000e-02);double(1)]')  Offsets=str2num('[double(0);double(0);double(0);double(0)]')  Minimums=str2num('[double(-300);double(0);double(-300);double(-Inf)]')  Maximums=str2num('[double(300);double(7);double(300);double(Inf)]')  ApplyMinMax=off
      settings: AttributesFormatString=<CANdbFile = %<CANdbFile>>  SourceProductName=Simulink Real-Time  SourceProductBaseCode=XP  DataFormat=CANdb specified signals
  Signal Specification{,1..3} (4 alike) : SignalSpecification
  Terminator{2..5} (4 alike) : Terminator
  HEVCtrl_Regen_brake_torque_available : Outport
  HEVCtrl_Regen_brake_torque_actual : Outport  Port=2
  VMCtrl_BrakeForceStatus : Outport  Port=3
  VMCtrl_BrakeForceCmnd : Outport  Port=4
  wires:
  BrakeCtrl_VehCAN Unpack2/3 -> Terminator2/1
  BrakeCtrl_VehCAN Unpack/3 -> Terminator4/1
  BrakeCtrl_VehCAN Unpack2/4 -> Terminator3/1
  BrakeCtrl_VehCAN Unpack/4 -> Terminator5/1
  BrakeCtrl_VehCAN Unpack2/1 -> Signal Specification2/1  "VehCAN_VMCtrl_BrakeForceCmnd"
  BrakeCtrl_VehCAN Unpack/2 -> Signal Specification1/1  "VehCAN_HEVCtrl_Regen_brake_torque_available"
  VehCAN_Msg/1 -> BrakeCtrl_VehCAN Unpack2/1, BrakeCtrl_VehCAN Unpack/1
  BrakeCtrl_VehCAN Unpack2/2 -> Signal Specification3/1  "VehCAN_VMCtrl_BrakeForceStatus"
  BrakeCtrl_VehCAN Unpack/1 -> Signal Specification/1  "VehCAN_HEVCtrl_Regen_brake_torque_actual"
  Signal Specification/1 -> HEVCtrl_Regen_brake_torque_actual/1  "HEVCtrl_Regen_brake_torque_actual"
  Signal Specification1/1 -> HEVCtrl_Regen_brake_torque_available/1  "HEVCtrl_Regen_brake_torque_available"
  Signal Specification2/1 -> VMCtrl_BrakeForceCmnd/1  "VMCtrl_BrakeForceCmnd"
  Signal Specification3/1 -> VMCtrl_BrakeForceStatus/1  "VMCtrl_BrakeForceStatus"

== system HEV_Simu_V1_1_RT/Controller/CtrlStrct_VNT_Level_2/VNT_Level_2_CAN/Engine_Ctrl/EngineCtrl_PwtrCAN_Rx/EngineCtrl_PwtrCAN_Receive_10ms ==
  PwtrCAN_Msg : Inport
  function : TriggerPort  TriggerType=function-call  VariantControl=Variant
  EngineCtrl_PwtrCAN Unpack : canmsglib/CAN Unpack  CANdbFile=HEV_CANDB.dbc  MsgList=HEV_Ctrl_PwtrCAN_Tx_1  MsgName=HEV_Ctrl_PwtrCAN_Tx_1  MsgIDType=Extended (29-bit identifier)  MsgIdentifier=218046594  MsgLength=8  SignalInfo=HEVCtrl_Engine_torque_request$0$16$1$1$1$0$1.562500e-02$0$-300$300$#HEVCtrl_Motor_torque_request$16$16$1$1$1$0$1.562500e-02$0$-300$300$#HEVCtrl_Regen_brake_torque_actua$48$16$1$1$1$0$6.250000e-02$0$-300$3000$#HEVCtrl_Regen_brake_torque_avail$32$16$1$1$1$0$6.250000e-02$0$-300$3000$#  NSignals=4  IDPort=off  TimestampPort=off  ErrorPort=off  RemotePort=off  LengthPort=off  StatusPort=off  StartBits=str2num('[int32(0);int32(16);int32(48);int32(32)]')  SignalSizes=str2num('[int32(16);int32(16);int32(16);int32(16)]')  ByteOrders=str2num('[int32(1);int32(1);int32(1);int32(1)]')  DataTypes=str2num('[int32(1);int32(1);int32(1);int32(1)]')  MultiplexTypes=str2num('[int32(1);int32(1);int32(1);int32(1)]')  MultiplexValues=str2num('[double(0);double(0);double(0);double(0)]')  Factors=str2num('[double(1.562500e-02);double(1.562500e-02);double(6.250000e-02);double(6.250000e-02)]')  Offsets=str2num('[double(0);double(0);double(0);double(0)]')  Minimums=str2num('[double(-300);double(-300);double(-300);double(-300)]')  Maximums=str2num('[double(300);double(300);double(3000);double(3000)]')  ApplyMinMax=off
      settings: AttributesFormatString=<CANdbFile = %<CANdbFile>>  SourceProductName=Simulink Real-Time  SourceProductBaseCode=XP  DataFormat=CANdb specified signals
  EngineCtrl_PwtrCAN Unpack2 : canmsglib/CAN Unpack  CANdbFile=HEV_CANDB.dbc  MsgList=HEV_Ctrl_PwtrCAN_Tx_2  MsgName=HEV_Ctrl_PwtrCAN_Tx_2  MsgIDType=Extended (29-bit identifier)  MsgIdentifier=218046850  MsgLength=8  SignalInfo=HEV_IdleStopCtrl_preparation_req$0$1$1$2$1$0$1$0$0$1$#HEV_IdleStopCtrl_request$1$1$1$2$1$0$1$0$0$1$#HEV_IdleStopCtrl_status$2$1$1$2$1$0$1$0$0$1$#  NSignals=3  IDPort=off  TimestampPort=off  ErrorPort=off  RemotePort=off  LengthPort=off  StatusPort=off  StartBits=str2num('[int32(0);int32(1);int32(2)]')  SignalSizes=str2num('[int32(1);int32(1);int32(1)]')  ByteOrders=str2num('[int32(1);int32(1);int32(1)]')  DataTypes=str2num('[int32(2);int32(2);int32(2)]')  MultiplexTypes=str2num('[int32(1);int32(1);int32(1)]')  MultiplexValues=str2num('[double(0);double(0);double(0)]')  Factors=str2num('[double(1);double(1);double(1)]')  Offsets=str2num('[double(0);double(0);double(0)]')  Minimums=str2num('[double(0);double(0);double(0)]')  Maximums=str2num('[double(1);double(1);double(1)]')  ApplyMinMax=off
      settings: AttributesFormatString=<CANdbFile = %<CANdbFile>>  SourceProductName=Simulink Real-Time  SourceProductBaseCode=XP  DataFormat=CANdb specified signals
  Signal Specification{,1..3} (4 alike) : SignalSpecification
  Terminator2 : Terminator
  Terminator3 : Terminator
  Terminator5 : Terminator
  HEVCtrl_Engine_torque_request : Outport
  HEVCtrl_IdleStop_preparation_request : Outport  Port=2
  HEVCtrl_IdleStop_request : Outport  Port=3
  HEVCtrl_IdleStop_status : Outport  Port=4
  wires:
  EngineCtrl_PwtrCAN Unpack2/3 -> Signal Specification3/1  "PwtrCAN_HEVCtrl_IdleStop_status"
  EngineCtrl_PwtrCAN Unpack/3 -> Terminator2/1
  EngineCtrl_PwtrCAN Unpack2/2 -> Signal Specification2/1  "PwtrCAN_HEVCtrl_IdleStop_request"
  EngineCtrl_PwtrCAN Unpack/1 -> Signal Specification/1  "PwtrCAN_HEVCtrl_Engine_torque_request"
  EngineCtrl_PwtrCAN Unpack/2 -> Terminator5/1
  EngineCtrl_PwtrCAN Unpack/4 -> Terminator3/1
  EngineCtrl_PwtrCAN Unpack2/1 -> Signal Specification1/1  "PwtrCAN_HEVCtrl_IdleStop_preparation_request"
  PwtrCAN_Msg/1 -> EngineCtrl_PwtrCAN Unpack2/1, EngineCtrl_PwtrCAN Unpack/1
  Signal Specification/1 -> HEVCtrl_Engine_torque_request/1  "HEVCtrl_Engine_torque_request"
  Signal Specification1/1 -> HEVCtrl_IdleStop_preparation_request/1  "HEVCtrl_IdleStop_preparation_request"
  Signal Specification2/1 -> HEVCtrl_IdleStop_request/1  "HEVCtrl_IdleStop_request"
  Signal Specification3/1 -> HEVCtrl_IdleStop_status/1  "HEVCtrl_IdleStop_status"

== system HEV_Simu_V1_1_RT/Controller/CtrlStrct_VNT_Level_2/VNT_Level_2_CAN/Gateway/Gateway PwtrCAN/Gateway_InfoCAN_Receive_100ms ==
  InfoCAN_Msg : Inport
  function : TriggerPort  TriggerType=function-call  VariantControl=Variant
  Gateway InfoCAN Unpack : canmsglib/CAN Unpack  CANdbFile=HEV_CANDB.dbc  MsgList=NAVI_InfoCAN_Tx  MsgName=NAVI_InfoCAN_Tx  MsgIDType=Extended (29-bit identifier)  MsgIdentifier=218083356  MsgLength=8  SignalInfo=NAVI_Home_around_status$16$16$1$2$1$0$1$0$0$65535$#NAVI_Road_information$0$16$1$2$1$0$1$0$0$65535$#  NSignals=2  IDPort=off  TimestampPort=off  ErrorPort=off  RemotePort=off  LengthPort=off  StatusPort=off  StartBits=str2num('[int32(16);int32(0)]')  SignalSizes=str2num('[int32(16);int32(16)]')  ByteOrders=str2num('[int32(1);int32(1)]')  DataTypes=str2num('[int32(2);int32(2)]')  MultiplexTypes=str2num('[int32(1);int32(1)]')  MultiplexValues=str2num('[double(0);double(0)]')  Factors=str2num('[double(1);double(1)]')  Offsets=str2num('[double(0);double(0)]')  Minimums=str2num('[double(0);double(0)]')  Maximums=str2num('[double(65535);double(65535)]')  ApplyMinMax=off
      settings: AttributesFormatString=<CANdbFile = %<CANdbFile>>  SourceProductName=Simulink Real-Time  SourceProductBaseCode=XP  DataFormat=CANdb specified signals
  Terminator : Terminator
  NAVI_Home_around_status : Outport
  wires:
  Gateway InfoCAN Unpack/2 -> Terminator/1
  Gateway InfoCAN Unpack/1 -> NAVI_Home_around_status/1  "InfoCAN_NAVI_Home_around_status"
  InfoCAN_Msg/1 -> Gateway InfoCAN Unpack/1

== system HEV_Simu_V1_1_RT/Controller/CtrlStrct_VNT_Level_2/VNT_Level_2_CAN/Gateway/Gateway PwtrCAN/Gateway_VehCAN_Receive_10ms ==
  VehCAN_Msg : Inport
  function : TriggerPort  TriggerType=function-call  VariantControl=Variant
  Gateway_VehCAN Unpack : canmsglib/CAN Unpack  CANdbFile=HEV_CANDB.dbc  MsgList=VM_Ctrl_VehCAN_Tx  MsgName=VM_Ctrl_VehCAN_Tx  MsgIDType=Extended (29-bit identifier)  MsgIdentifier=218091654  MsgLength=8  SignalInfo=VMCtrl_BrakeTorqCmnd$32$16$1$1$1$0$1.000000e-02$0$-300$300$#VMCtrl_BrakeTorqStatus$24$8$1$2$1$0$1$0$0$7$#VMCtrl_PropTorqCmnd$8$16$1$1$1$0$1.000000e-02$0$-300$300$#VMCtrl_PropTorqStatus$0$8$1$2$1$0$1$0$-Inf$Inf$#  NSignals=4  IDPort=off  TimestampPort=off  ErrorPort=off  RemotePort=off  LengthPort=off  StatusPort=off  StartBits=str2num('[int32(32);int32(24);int32(8);int32(0)]')  SignalSizes=str2num('[int32(16);int32(8);int32(16);int32(8)]')  ByteOrders=str2num('[int32(1);int32(1);int32(1);int32(1)]')  DataTypes=str2num('[int32(1);int32(2);int32(1);int32(2)]')  MultiplexTypes=str2num('[int32(1);int32(1);int32(1);int32(1)]')  MultiplexValues=str2num('[double(0);double(0);double(0);double(0)]')  Factors=str2num('[double(1.000000e-02);double(1);double(1.000000e-02);double(1)]')  Offsets=str2num('[double(0);double(0);double(0);double(0)]')  Minimums=str2num('[double(-300);double(0);double(-300);double(-Inf)]')  Maximums=str2num('[double(300);double(7);double(300);double(Inf)]')  ApplyMinMax=off
      settings: AttributesFormatString=<CANdbFile = %<CANdbFile>>  SourceProductName=Simulink Real-Time  SourceProductBaseCode=XP  DataFormat=CANdb specified signals
  Gateway_VehCAN Unpack3 : canmsglib/CAN Unpack  CANdbFile=HEV_CANDB.dbc  MsgList=BrakeCtrl_VehCAN_Tx  MsgName=BrakeCtrl_VehCAN_Tx  MsgIDType=Extended (29-bit identifier)  MsgIdentifier=218062859  MsgLength=8  SignalInfo=BrkCtrl_Regen_brake_torque_reque$16$16$1$1$1$0$1.000000e-02$0$-300$300$#BrkCtrl_Vehicle_speed$0$16$1$2$1$0$1.000000e-01$0$0$180$#  NSignals=2  IDPort=off  TimestampPort=off  ErrorPort=off  RemotePort=off  LengthPort=off  StatusPort=off  StartBits=str2num('[int32(16);int32(0)]')  SignalSizes=str2num('[int32(16);int32(16)]')  ByteOrders=str2num('[int32(1);int32(1)]')  DataTypes=str2num('[int32(1);int32(2)]')  MultiplexTypes=str2num('[int32(1);int32(1)]')  MultiplexValues=str2num('[double(0);double(0)]')  Factors=str2num('[double(1.000000e-02);double(1.000000e-01)]')  Offsets=str2num('[double(0);double(0)]')  Minimums=str2num('[double(-300);double(0)]')  Maximums=str2num('[double(300);double(180)]')  ApplyMinMax=off
      settings: AttributesFormatString=<CANdbFile = %<CANdbFile>>  SourceProductName=Simulink Real-Time  SourceProductBaseCode=XP  DataFormat=CANdb specified signals
  Terminator1 : Terminator
  Terminator2 : Terminator
  VMCtrl_PropTorqCmnd : Outport
  VMCtrl_PropTorqStatus : Outport  Port=2
  BrkCtrl_Regen_brake_torque_request : Outport  Port=3
  BrkCtrl_Vehicle_speed : Outport  Port=4
  wires:
  Gateway_VehCAN Unpack/3 -> VMCtrl_PropTorqCmnd/1  "VehCAN_VMCtrl_PropTorqCmnd"
  VehCAN_Msg/1 -> Gateway_VehCAN Unpack3/1, Gateway_VehCAN Unpack/1
  Gateway_VehCAN Unpack3/2 -> BrkCtrl_Vehicle_speed/1  "VehCAN_BrkCtrl_Vehicle_speed"
  Gateway_VehCAN Unpack/1 -> Terminator1/1
  Gateway_VehCAN Unpack/2 -> Terminator2/1
  Gateway_VehCAN Unpack/4 -> VMCtrl_PropTorqStatus/1  "VehCAN_VMCtrl_PropTorqStatus"
  Gateway_VehCAN Unpack3/1 -> BrkCtrl_Regen_brake_torque_request/1  "VehCAN_BrkCtrl_Regen_brake_torque_request"

== system HEV_Simu_V1_1_RT/Controller/CtrlStrct_VNT_Level_2/VNT_Level_2_CAN/Gateway/Gateway PwtrCAN/Gateway_VehCAN_Receive_50ms ==
  VehCAN_Msg : Inport
  function : TriggerPort  TriggerType=function-call  VariantControl=Variant
  Gateway_VehCAN Unpack2 : canmsglib/CAN Unpack  CANdbFile=HEV_CANDB.dbc  MsgList=BodyCtrl_VehCAN_Tx  MsgName=BodyCtrl_VehCAN_Tx  MsgIDType=Extended (29-bit identifier)  MsgIdentifier=218079272  MsgLength=8  SignalInfo=BdyCtrl_Door_open_flag$1$1$1$2$1$0$1$0$0$1$#BdyCtrl_Engine_hood_open_flag$1$1$1$2$1$0$1$0$0$1$#BdyCtrl_Idlestop_cancel$0$1$1$2$1$0$1$0$0$1$#  NSignals=3  IDPort=off  TimestampPort=off  ErrorPort=off  RemotePort=off  LengthPort=off  StatusPort=off  StartBits=str2num('[int32(1);int32(1);int32(0)]')  SignalSizes=str2num('[int32(1);int32(1);int32(1)]')  ByteOrders=str2num('[int32(1);int32(1);int32(1)]')  DataTypes=str2num('[int32(2);int32(2);int32(2)]')  MultiplexTypes=str2num('[int32(1);int32(1);int32(1)]')  MultiplexValues=str2num('[double(0);double(0);double(0)]')  Factors=str2num('[double(1);double(1);double(1)]')  Offsets=str2num('[double(0);double(0);double(0)]')  Minimums=str2num('[double(0);double(0);double(0)]')  Maximums=str2num('[double(1);double(1);double(1)]')  ApplyMinMax=off
      settings: AttributesFormatString=<CANdbFile = %<CANdbFile>>  SourceProductName=Simulink Real-Time  SourceProductBaseCode=XP  DataFormat=CANdb specified signals
  Gateway_VehCAN Unpack4 : canmsglib/CAN Unpack  CANdbFile=HEV_CANDB.dbc  MsgList=HVAC_Ctrl_VehCAN_Tx  MsgName=HVAC_Ctrl_VehCAN_Tx  MsgIDType=Extended (29-bit identifier)  MsgIdentifier=218095751  MsgLength=8  SignalInfo=HVAC_Ctrl_Idlestop_cancel$1$1$1$2$1$0$1$0$0$1$#HVAC_Ctrl_Idlestop_enbl$0$1$1$2$1$0$1$0$0$1$#  NSignals=2  IDPort=off  TimestampPort=off  ErrorPort=off  RemotePort=off  LengthPort=off  StatusPort=off  StartBits=str2num('[int32(1);int32(0)]')  SignalSizes=str2num('[int32(1);int32(1)]')  ByteOrders=str2num('[int32(1);int32(1)]')  DataTypes=str2num('[int32(2);int32(2)]')  MultiplexTypes=str2num('[int32(1);int32(1)]')  MultiplexValues=str2num('[double(0);double(0)]')  Factors=str2num('[double(1);double(1)]')  Offsets=str2num('[double(0);double(0)]')  Minimums=str2num('[double(0);double(0)]')  Maximums=str2num('[double(1);double(1)]')  ApplyMinMax=off
      settings: AttributesFormatString=<CANdbFile = %<CANdbFile>>  SourceProductName=Simulink Real-Time  SourceProductBaseCode=XP  DataFormat=CANdb specified signals
  Gateway_VehCAN Unpack5 : canmsglib/CAN Unpack  CANdbFile=HEV_CANDB.dbc  MsgList=SteerCtrl_VehCAN_Tx  MsgName=SteerCtrl_VehCAN_Tx  MsgIDType=Extended (29-bit identifier)  MsgIdentifier=218066963  MsgLength=8  SignalInfo=StrgCtrl_Steer_angle$0$16$1$1$1$0$3.125000e-02$0$-720$720$#  NSignals=1  IDPort=off  TimestampPort=off  ErrorPort=off  RemotePort=off  LengthPort=off  StatusPort=off  StartBits=str2num('[int32(0)]')  SignalSizes=str2num('[int32(16)]')  ByteOrders=str2num('[int32(1)]')  DataTypes=str2num('[int32(1)]')  MultiplexTypes=str2num('[int32(1)]')  MultiplexValues=str2num('[double(0)]')  Factors=str2num('[double(3.125000e-02)]')  Offsets=str2num('[double(0)]')  Minimums=str2num('[double(-720)]')  Maximums=str2num('[double(720)]')  ApplyMinMax=off
      settings: AttributesFormatString=<CANdbFile = %<CANdbFile>>  SourceProductName=Simulink Real-Time  SourceProductBaseCode=XP  DataFormat=CANdb specified signals
  BdyCtrl_Door_open_flag : Outport
  BdyCtrl_Engine_hood_open_flag : Outport  Port=2
  BdyCtrl_Idlestop_cancel : Outport  Port=3
  HVAC_Ctrl_Idlestop_cancel : Outport  Port=4
  HVAC_Ctrl_Idlestop_enbl : Outport  Port=5
  StrgCtrl_Steer_angle : Outport  Port=6
  wires:
  Gateway_VehCAN Unpack5/1 -> StrgCtrl_Steer_angle/1  "VehCAN_StrgCtrl_Steer_angle"
  VehCAN_Msg/1 -> Gateway_VehCAN Unpack5/1, Gateway_VehCAN Unpack4/1, Gateway_VehCAN Unpack2/1
  Gateway_VehCAN Unpack4/1 -> HVAC_Ctrl_Idlestop_cancel/1  "VehCAN_HVAC_Ctrl_Idlestop_cancel"
  Gateway_VehCAN Unpack4/2 -> HVAC_Ctrl_Idlestop_enbl/1  "VehCAN_HVAC_Ctrl_Idlestop_enbl"
  Gateway_VehCAN Unpack2/1 -> BdyCtrl_Door_open_flag/1  "VehCAN_BdyCtrl_Door_open_flag"
  Gateway_VehCAN Unpack2/3 -> BdyCtrl_Idlestop_cancel/1  "VehCAN_BdyCtrl_Idlestop_cancel"
  Gateway_VehCAN Unpack2/2 -> BdyCtrl_Engine_hood_open_flag/1  "VehCAN_BdyCtrl_Engine_hood_open_flag"
